simulink library "customLib"  (R2021b)
settings: Solver=VariableStepAuto  StartTime=0.0  StopTime=10.0  RelTol=1e-3
undefined symbols (not defined in the file or in its folder): D1, Delta
libraries: eeGeneralControl x7, spsParallelRLCBranchLib x6, spsSeriesRLCBranchLib x3, slpidlib x2, spsThreePhaseTransformerTwoWindingsLib x1
settings Model: Creator=ah4430  LastModifiedBy=ah4430

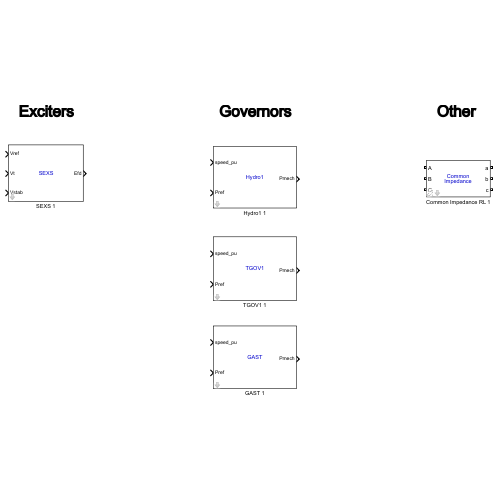
[thumbnail: Simulink's stored preview of the top-level diagram]
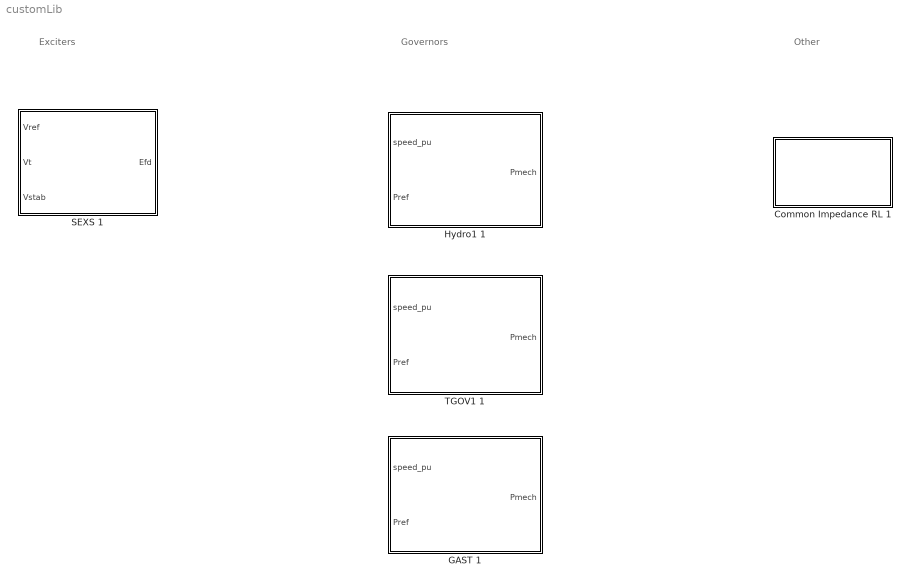
== system customLib ==
  note: Exciters
  note: Governors
  note: Other
  Common Impedance RL 1 : Subsystem  AncestorBlock=customLib/Common Impedance 1  mask{R=0.001, L=0, C=0, Ui=0, Ri=1e3, Li=1e-3, Uj=0, Rj=1e3, Lj=1e-3, Winding1Connection=Delta (D1), Winding2Connection=Delta (D1), ConnectionVariant=abc}
      mask prompts: R "Resistance [Ohm]"; L "Inductance [H]"; C "Capacitance [F]"; Ui "Voltage i [V]"; Ri "Resistance i [Ohm]"; Li "Inductance i [H]"; Uj "Voltage j [V]"; Rj "Resistance j [Ohm]"; Lj "Inductance j [H]"; Winding1Connection "Winding 1 connection (ABC terminals):"; Winding2Connection "Winding 2 connection (abc terminals):"; ConnectionVariant "Connection (abc, bca, cab)"
      mask TypeOptions Winding1Connection: Transformer/Winding1Connection
      mask TypeOptions Winding2Connection: Transformer/Winding2Connection
      mask TypeOptions ConnectionVariant: Connection/LabelModeActiveChoice
      mask Display: color('blue');disp('Common\nImpedance')
  GAST 1 : Subsystem  mask{R=0.05, T_1=0.2, T_2=0.2, T_3=1, A_T=0.5, K_T=1, Vmax=1.1, Vmin=0, DTurb=0}
      mask prompts: R "Permanent droop R (pu)"; T_1 "Governor mechanism time constant T_1 (s)"; T_2 "Turbine power time constant T_2 (s)"; T_3 "Turbine exhaust temperature time constant T_3 (s)"; A_T "Ambient temperature load limit A_T (pu)"; K_T "Temperature limiter gain K_T (pu)"; Vmax "Maximum turbine power Vmax (pu)"; Vmin "Minimum turbine power Vmin (pu)"; DTurb "Turbine damping factor DTurb (pu)"
      mask Display: color('blue');disp('GAST')
  Hydro1 1 : Subsystem  mask{Rt=0.3, TR=5, TF=0.05, TG=0.5, TW=1, AT=10, DT=0.5, QNL=0.08, Rp=0.29, Gmin=0, Gmax=1, Velm=0.2}
      mask prompts: Rt "Temporary droop Rt (pu)"; TR "Governor time constant TR (s)"; TF "Filter time constant TF (s)"; TG "Servo time constant TG (s)"; TW "Water starting time TW (s)"; AT "Turbine gain AT (pu)"; DT "Turbine damping factor DT (pu)"; QNL "No load flow QNL (pu)"; Rp "Permanent droop Rp (pu)"; Gmin "Minimum gate limit Gmin (pu)"; Gmax "Maximum gate limit Gmax (pu)"; Velm "Gate velocity limit Velm (pu)"
      mask Display: color('blue');disp('Hydro1')
  SEXS 1 : Subsystem  mask{TA=0, TB=0, K=0, TE=0, Emin=0, Emax=0}
      mask prompts: TA "Filter lead time constant TA (s)"; TB "Filter lag time constant TB (s)"; K "Controller gain K (pu)"; TE "Exciter time constant TE (s)"; Emin "Exciter minimum output Emin (pu)"; Emax "Exciter maximum output Emax (pu)"
      mask Display: color('blue');disp('SEXS')
  TGOV1 1 : Subsystem  mask(Governor TGOV1){R=0.05, T_1=0.2, Vmax=1.2, Vmin=0, T_2=1, T_3=3, Dt=0}
      mask prompts: R "Permanent droop R (pu)"; T_1 "Steam bowl time constant T_1 (s)"; Vmax "Maximum valve position Vmax (pu)"; Vmin "Minimum valve position Vmin (pu)"; T_2 "Time constant of high-pressure fraction T_2 (s)"; T_3 "Reheater time constant T_3 (s)"; Dt "Turbine damping coefficient Dt (pu)"
      mask help: Implements a TGOV1 governor.
      mask Display: color('blue');disp('TGOV1')

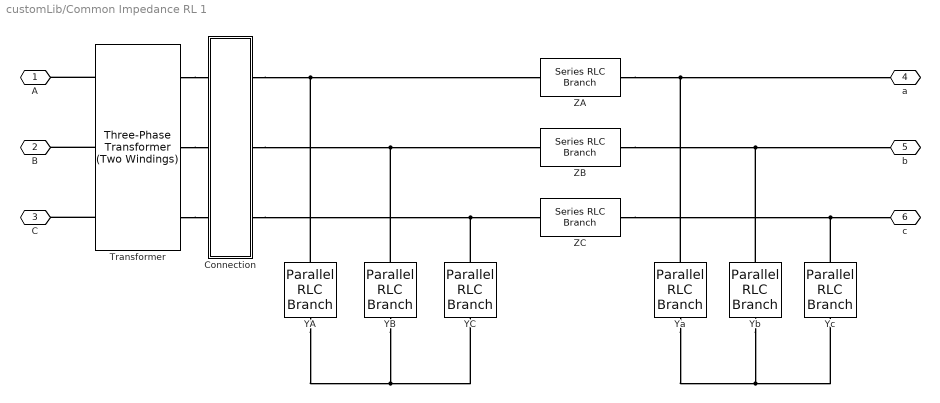
== system customLib/Common Impedance RL 1 ==
  Connection : Subsystem  Variant=on  VariantControlMode=label  LabelModeActiveChoice=abc
  Transformer : spsThreePhaseTransformerTwoWindingsLib/Three-Phase Transformer (Two Windings)  VariantControl=(default)  Winding1Connection=Delta (D1)  Winding2Connection=Delta (D1)  CoreType=Three single-phase transformers  SetSaturation=off  Hysteresis=off  DataFile='hysteresis'  SetInitialFlux=off  Measurements=None  UNITS=pu  NominalPower=[ 1e12 , 60 ]  Winding1=[Ui 1e-7 0]  Winding2=[Uj 1e-7 0]  Rm=1e7  Lm=1e7  L0=NaN  Saturation=[NaN NaN;NaN NaN;NaN NaN]  InitialFluxes=[NaN NaN NaN]  BreakLoop=off  DiscreteSolver=Trapezoidal iterative  DataType=off  TransfoNumber=1
  YA : spsParallelRLCBranchLib/Parallel RLC Branch  LConnTagsString=a  RConnTagsString=__new0  BranchType=RL  Resistance=Ri  Inductance=Li  SetiL0=off  InitialCurrent=0  Capacitance=1e-6  Setx0=off  InitialVoltage=0  Measurements=None
  YB : spsParallelRLCBranchLib/Parallel RLC Branch  LConnTagsString=a  RConnTagsString=__new0  BranchType=RL  Resistance=Ri  Inductance=Li  SetiL0=off  InitialCurrent=0  Capacitance=1e-6  Setx0=off  InitialVoltage=0  Measurements=None
  YC : spsParallelRLCBranchLib/Parallel RLC Branch  LConnTagsString=a  RConnTagsString=__new0  BranchType=RL  Resistance=Ri  Inductance=Li  SetiL0=off  InitialCurrent=0  Capacitance=1e-6  Setx0=off  InitialVoltage=0  Measurements=None
  Ya : spsParallelRLCBranchLib/Parallel RLC Branch  LConnTagsString=a  RConnTagsString=__new0  BranchType=RL  Resistance=Rj  Inductance=Lj  SetiL0=off  InitialCurrent=0  Capacitance=1e-6  Setx0=off  InitialVoltage=0  Measurements=None
  Yb : spsParallelRLCBranchLib/Parallel RLC Branch  LConnTagsString=a  RConnTagsString=__new0  BranchType=RL  Resistance=Rj  Inductance=Lj  SetiL0=off  InitialCurrent=0  Capacitance=1e-6  Setx0=off  InitialVoltage=0  Measurements=None
  Yc : spsParallelRLCBranchLib/Parallel RLC Branch  LConnTagsString=a  RConnTagsString=__new0  BranchType=RL  Resistance=Rj  Inductance=Lj  SetiL0=off  InitialCurrent=0  Capacitance=1e-6  Setx0=off  InitialVoltage=0  Measurements=None
  ZA : spsSeriesRLCBranchLib/Series RLC Branch  LConnTagsString=__new0  RConnTagsString=__new0  BranchType=RL  Resistance=R  Inductance=L  SetiL0=off  InitialCurrent=0  Capacitance=C  Setx0=off  InitialVoltage=0  Measurements=None
  ZB : spsSeriesRLCBranchLib/Series RLC Branch  LConnTagsString=__new0  RConnTagsString=__new0  BranchType=RL  Resistance=R  Inductance=L  SetiL0=off  InitialCurrent=0  Capacitance=C  Setx0=off  InitialVoltage=0  Measurements=None
  ZC : spsSeriesRLCBranchLib/Series RLC Branch  LConnTagsString=__new0  RConnTagsString=__new0  BranchType=RL  Resistance=R  Inductance=L  SetiL0=off  InitialCurrent=0  Capacitance=C  Setx0=off  InitialVoltage=0  Measurements=None
  A : PMIOPort  Side=Left
  B : PMIOPort  Port=2  Side=Left
  C : PMIOPort  Port=3  Side=Left
  a : PMIOPort  Port=4  Side=Right
  b : PMIOPort  Port=5  Side=Right
  c : PMIOPort  Port=6  Side=Right
  connections:
  YA/LConn1 -- ZA/LConn1 -- Connection/LConn1
  YC/LConn1 -- ZC/LConn1 -- Connection/LConn3
  YB/LConn1 -- ZB/LConn1 -- Connection/LConn2
  Ya/LConn1 -- ZA/RConn1 -- a/RConn1
  Yb/LConn1 -- ZB/RConn1 -- b/RConn1
  Yc/LConn1 -- ZC/RConn1 -- c/RConn1
  Transformer/LConn1 -- A/RConn1
  Transformer/LConn2 -- B/RConn1
  Transformer/LConn3 -- C/RConn1
  Ya/RConn1 -- Yb/RConn1 -- Yc/RConn1
  Transformer/RConn1 -- Connection/RConn1
  Transformer/RConn2 -- Connection/RConn2
  Transformer/RConn3 -- Connection/RConn3
  YB/RConn1 -- YC/RConn1 -- YA/RConn1

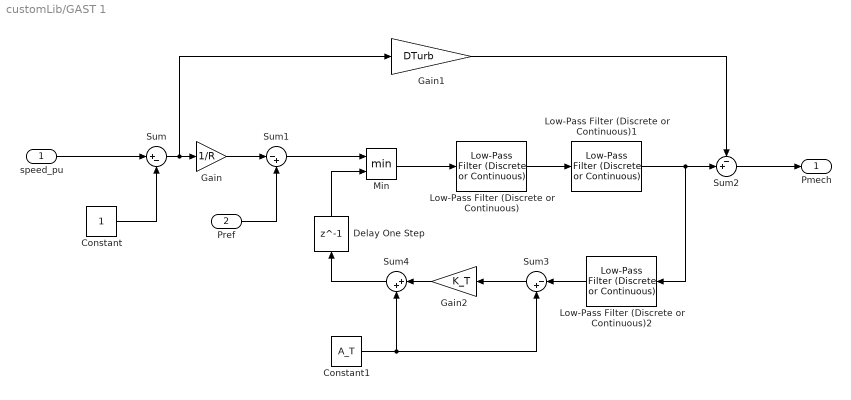
== system customLib/GAST 1 ==
  speed_pu : Inport
  Pref : Inport  Port=2
  Constant : Constant
  Constant1 : Constant  Value=A_T
  Delay One Step : Delay  DelayLength=1
  Gain : Gain  Gain=1/R
  Gain1 : Gain  Gain=DTurb
  Gain2 : Gain  Gain=K_T
  Low-Pass Filter (Discrete or Continuous) : eeGeneralControl/Low-Pass Filter (Discrete or Continuous)  K=1  T=T_1  B=Vmax  A=Vmin  init_option=Inherited from block input  x0=0  Ts=-1
  Low-Pass Filter (Discrete or Continuous)1 : eeGeneralControl/Low-Pass Filter (Discrete or Continuous)  K=1  T=T_2  B=inf  A=-inf  init_option=Inherited from block input  x0=0  Ts=-1
  Low-Pass Filter (Discrete or Continuous)2 : eeGeneralControl/Low-Pass Filter (Discrete or Continuous)  K=1  T=T_3  B=inf  A=-inf  init_option=Inherited from block input  x0=0  Ts=-1
  Min : MinMax  Inputs=2
  Sum : Sum  Inputs=|+-
  Sum1 : Sum  Inputs=|-+
  Sum2 : Sum  Inputs=-+|
  Sum3 : Sum  Inputs=|-+
  Sum4 : Sum  Inputs=|++
  Pmech : Outport
  wires:
  speed_pu/1 -> Sum/1
  Constant/1 -> Sum/2
  Sum/1 -> Gain1/1, Gain/1
  Gain/1 -> Sum1/1
  Pref/1 -> Sum1/2
  Sum1/1 -> Min/1
  Min/1 -> Low-Pass Filter (Discrete or Continuous)/1
  Low-Pass Filter (Discrete or Continuous)/1 -> Low-Pass Filter (Discrete or Continuous)1/1
  Low-Pass Filter (Discrete or Continuous)1/1 -> Low-Pass Filter (Discrete or Continuous)2/1, Sum2/2
  Gain1/1 -> Sum2/1
  Sum2/1 -> Pmech/1
  Low-Pass Filter (Discrete or Continuous)2/1 -> Sum3/1
  Constant1/1 -> Sum4/2, Sum3/2
  Sum3/1 -> Gain2/1
  Gain2/1 -> Sum4/1
  Sum4/1 -> Delay One Step/1
  Delay One Step/1 -> Min/2

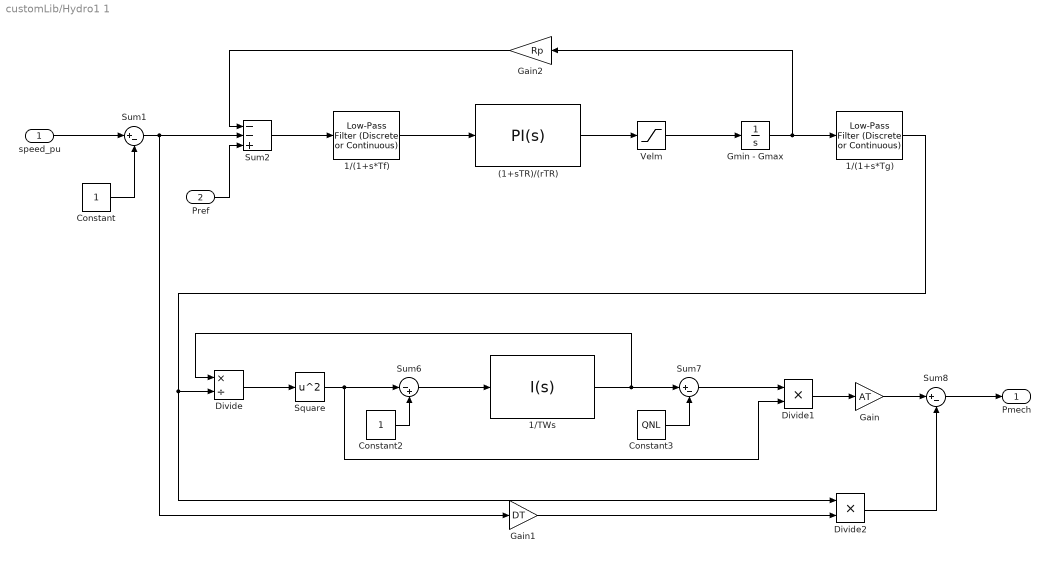
== system customLib/Hydro1 1 ==
  speed_pu : Inport
  Pref : Inport  Port=2
  (1+sTR)/(rTR) : slpidlib/PID Controller  Controller=PI  Form=Parallel  TimeDomain=Continuous-time  UseExternalTs=off  SampleTime=-1  IntegratorMethod=Forward Euler  FilterMethod=Forward Euler  ControllerParametersSource=internal  P=1/Rt  I=1/(Rt*TR)  D=0  UseFilter=on  N=100  TunerSelectOption=Transfer Function Based (PID Tuner App)  InitialConditionSource=internal  InitialConditionForIntegrator=0  InitialConditionForFilter=0  DifferentiatorICPrevScaledInput=0  ExternalReset=none  TrackingMode=off  Kt=1  LimitOutput=on  SatLimitsSource=internal  UpperSaturationLimit=Gmax  LowerSaturationLimit=Gmin  LinearizeAsGain=on  AntiWindupMode=none  Kb=1  POutMin=[]  POutMax=[]  IOutMin=[]  IOutMax=[]  DOutMin=[]  DOutMax=[]  NOutMin=[]  NOutMax=[]  SumOutMin=[]  SumOutMax=[]  SaturationOutMin=[]  SaturationOutMax=[]  PParamMin=[]  PParamMax=[]  IParamMin=[]  IParamMax=[]  DParamMin=[]  DParamMax=[]  NParamMin=[]  NParamMax=[]  KbParamMin=[]  KbParamMax=[]  KtParamMin=[]  KtParamMax=[]  KbOutMin=[]  KbOutMax=[]  KtOutMin=[]  KtOutMax=[]  IntegratorOutMin=[]  IntegratorOutMax=[]  FilterOutMin=[]  FilterOutMax=[]  SumI1OutMin=[]  SumI1OutMax=[]  SumI2OutMin=[]  SumI2OutMax=[]  SumI3OutMin=[]  SumI3OutMax=[]  SumI4OutMin=[]  SumI4OutMax=[]  SumDOutMin=[]  SumDOutMax=[]  DifferentiatorOutMin=[]  DifferentiatorOutMax=[]  FilterDiffOutCoefMin=[]  FilterDiffOutCoefMax=[]  ReciprocalOutMin=[]  ReciprocalOutMax=[]  SumDenOutMin=[]  SumDenOutMax=[]  SumNumOutMin=[]  SumNumOutMax=[]  DivideOutMin=[]  DivideOutMax=[]  UdiffTsProdOutMin=[]  UdiffTsProdOutMax=[]  NTsProdOutMin=[]  NTsProdOutMax=[]  UintegralTsProdOutMin=[]  UintegralTsProdOutMax=[]  UngainTsProdOutMin=[]  UngainTsProdOutMax=[]  FilterDenConstantOutDataTypeStr=Inherit: Inherit via back propagation  FilterDenConstantOutMin=[]  FilterDenConstantOutMax=[]  PCopyOutDataTypeStr=Inherit: Inherit via back propagation  PCopyOutMin=[]  PCopyOutMax=[]  NCopyOutDataTypeStr=Inherit: Inherit via back propagation  NCopyOutMin=[]  NCopyOutMax=[]  IntegratorContinuousStateAttributes=''  IntegratorStateMustResolveToSignalObject=off  IntegratorRTWStateStorageClass=Auto  FilterContinuousStateAttributes=''  FilterStateMustResolveToSignalObject=off  FilterRTWStateStorageClass=Auto  ParallelPVariant=InternalParameters  IdealPVariant=Disabled  IVariant=InternalParameters  DVariant=Disabled  IntegratorVariant=Continuous  SatVariant=Enabled  AWVariant=Passthrough  PCopyVariant=Disabled  TRVariant=Disabled  FdbkBlocksVariant=Forward  IdealPFdbkVariant=Disabled  SatFdbkVariant=Disabled  DerivativeFilterVariant=Disabled  NVariant=Disabled  NCopyVariant=Disabled_SignalSpec  FilterICVariant=Disabled  IntegratorICVariant=InternalICs  ExternalResetVariant=Disabled  TRSumVariant=Passthrough  SumFdbkVariant=Disabled  SumVariant=Sum_PI  TsampFilterVariant=InternalTs  TsampNgainVariant=Passthrough  TsampIntegralVariant=Passthrough  ExternalSaturationOutDataTypeStr=Inherit: Same as second input
  1/(1+s*Tf) : eeGeneralControl/Low-Pass Filter (Discrete or Continuous)  K=1  T=TF  B=inf  A=-inf  init_option=Inherited from block input  x0=0  Ts=-1
  1/(1+s*Tg) : eeGeneralControl/Low-Pass Filter (Discrete or Continuous)  K=1  T=TG  B=inf  A=-inf  init_option=Inherited from block input  x0=0  Ts=-1
  1/TWs : slpidlib/PID Controller  Controller=I  Form=Parallel  TimeDomain=Continuous-time  UseExternalTs=off  SampleTime=-1  IntegratorMethod=Forward Euler  FilterMethod=Forward Euler  ControllerParametersSource=internal  P=1  I=1/TW  D=0  UseFilter=on  N=100  TunerSelectOption=Transfer Function Based (PID Tuner App)  InitialConditionSource=internal  InitialConditionForIntegrator=0  InitialConditionForFilter=0  DifferentiatorICPrevScaledInput=0  ExternalReset=none  TrackingMode=off  Kt=1  LimitOutput=on  SatLimitsSource=internal  UpperSaturationLimit=Gmax  LowerSaturationLimit=Gmin  LinearizeAsGain=on  AntiWindupMode=none  Kb=1  POutMin=[]  POutMax=[]  IOutMin=[]  IOutMax=[]  DOutMin=[]  DOutMax=[]  NOutMin=[]  NOutMax=[]  SumOutMin=[]  SumOutMax=[]  SaturationOutMin=[]  SaturationOutMax=[]  PParamMin=[]  PParamMax=[]  IParamMin=[]  IParamMax=[]  DParamMin=[]  DParamMax=[]  NParamMin=[]  NParamMax=[]  KbParamMin=[]  KbParamMax=[]  KtParamMin=[]  KtParamMax=[]  KbOutMin=[]  KbOutMax=[]  KtOutMin=[]  KtOutMax=[]  IntegratorOutMin=[]  IntegratorOutMax=[]  FilterOutMin=[]  FilterOutMax=[]  SumI1OutMin=[]  SumI1OutMax=[]  SumI2OutMin=[]  SumI2OutMax=[]  SumI3OutMin=[]  SumI3OutMax=[]  SumI4OutMin=[]  SumI4OutMax=[]  SumDOutMin=[]  SumDOutMax=[]  DifferentiatorOutMin=[]  DifferentiatorOutMax=[]  FilterDiffOutCoefMin=[]  FilterDiffOutCoefMax=[]  ReciprocalOutMin=[]  ReciprocalOutMax=[]  SumDenOutMin=[]  SumDenOutMax=[]  SumNumOutMin=[]  SumNumOutMax=[]  DivideOutMin=[]  DivideOutMax=[]  UdiffTsProdOutMin=[]  UdiffTsProdOutMax=[]  NTsProdOutMin=[]  NTsProdOutMax=[]  UintegralTsProdOutMin=[]  UintegralTsProdOutMax=[]  UngainTsProdOutMin=[]  UngainTsProdOutMax=[]  FilterDenConstantOutDataTypeStr=Inherit: Inherit via back propagation  FilterDenConstantOutMin=[]  FilterDenConstantOutMax=[]  PCopyOutDataTypeStr=Inherit: Inherit via back propagation  PCopyOutMin=[]  PCopyOutMax=[]  NCopyOutDataTypeStr=Inherit: Inherit via back propagation  NCopyOutMin=[]  NCopyOutMax=[]  IntegratorContinuousStateAttributes=''  IntegratorStateMustResolveToSignalObject=off  IntegratorRTWStateStorageClass=Auto  FilterContinuousStateAttributes=''  FilterStateMustResolveToSignalObject=off  FilterRTWStateStorageClass=Auto  ParallelPVariant=Disabled  IdealPVariant=Disabled  IVariant=InternalParameters  DVariant=Disabled  IntegratorVariant=Continuous  SatVariant=Enabled  AWVariant=Passthrough  PCopyVariant=Disabled  TRVariant=Disabled  FdbkBlocksVariant=Forward  IdealPFdbkVariant=Disabled  SatFdbkVariant=Disabled  DerivativeFilterVariant=Disabled  NVariant=Disabled  NCopyVariant=Disabled_SignalSpec  FilterICVariant=Disabled  IntegratorICVariant=InternalICs  ExternalResetVariant=Disabled  TRSumVariant=Passthrough  SumFdbkVariant=Disabled  SumVariant=Passthrough_I  TsampFilterVariant=InternalTs  TsampNgainVariant=Passthrough  TsampIntegralVariant=Passthrough  ExternalSaturationOutDataTypeStr=Inherit: Same as second input
  Constant : Constant
  Constant2 : Constant
  Constant3 : Constant  Value=QNL
  Divide : Product  Inputs=*/
  Divide1 : Product
  Divide2 : Product
  Gain : Gain  Gain=AT
  Gain1 : Gain  Gain=DT
  Gain2 : Gain  Gain=Rp
  Gmin - Gmax : Integrator  LimitOutput=on  UpperSaturationLimit=Gmax  LowerSaturationLimit=Gmin
  Square : Math  Operator=square  SaturateOnIntegerOverflow=on
  Sum1 : Sum  Inputs=|+-
  Sum2 : Sum  Inputs=--+
  Sum6 : Sum  Inputs=|-+
  Sum7 : Sum  Inputs=|+-
  Sum8 : Sum  Inputs=|+-
  Velm : Saturate  UpperLimit=Velm  LowerLimit=-1 * Velm
  Pmech : Outport
  wires:
  Constant/1 -> Sum1/2
  speed_pu/1 -> Sum1/1
  Pref/1 -> Sum2/3
  Sum1/1 -> Sum2/2, Gain1/1
  Sum2/1 -> 1/(1+s*Tf)/1
  (1+sTR)/(rTR)/1 -> Velm/1
  1/(1+s*Tf)/1 -> (1+sTR)/(rTR)/1
  Velm/1 -> Gmin - Gmax/1
  Gmin - Gmax/1 -> 1/(1+s*Tg)/1, Gain2/1
  Gain2/1 -> Sum2/1
  1/(1+s*Tg)/1 -> Divide2/1, Divide/2
  Divide/1 -> Square/1
  Constant2/1 -> Sum6/2
  Square/1 -> Divide1/2, Sum6/1
  Sum6/1 -> 1/TWs/1
  1/TWs/1 -> Divide/1, Sum7/1
  Constant3/1 -> Sum7/2
  Sum7/1 -> Divide1/1
  Divide1/1 -> Gain/1
  Gain/1 -> Sum8/1
  Divide2/1 -> Sum8/2
  Gain1/1 -> Divide2/2
  Sum8/1 -> Pmech/1

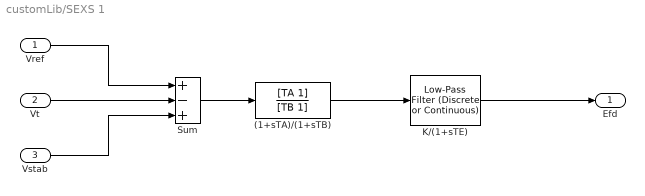
== system customLib/SEXS 1 ==
  Vref : Inport
  Vt : Inport  Port=2
  Vstab : Inport  Port=3
  (1+sTA)/(1+sTB) : TransferFcn  Numerator=[TA 1]  Denominator=[TB 1]
  K/(1+sTE) : eeGeneralControl/Low-Pass Filter (Discrete or Continuous)  K=K  T=TE  B=Emax  A=Emin  init_option=Inherited from block input  x0=0  Ts=-1
  Sum : Sum  Inputs=+-+
  Efd : Outport
  wires:
  Vref/1 -> Sum/1
  Vt/1 -> Sum/2
  Vstab/1 -> Sum/3
  Sum/1 -> (1+sTA)/(1+sTB)/1
  (1+sTA)/(1+sTB)/1 -> K/(1+sTE)/1
  K/(1+sTE)/1 -> Efd/1

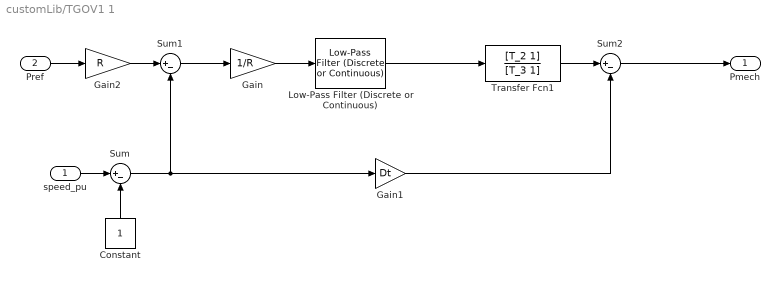
== system customLib/TGOV1 1 ==
  speed_pu : Inport
  Pref : Inport  Port=2
  Constant : Constant
  Gain : Gain  Gain=1/R
  Gain1 : Gain  Gain=Dt
  Gain2 : Gain  Gain=R
  Low-Pass Filter (Discrete or Continuous) : eeGeneralControl/Low-Pass Filter (Discrete or Continuous)  K=1  T=T_1  B=Vmax  A=Vmin  init_option=Inherited from block input  x0=0  Ts=-1
  Sum : Sum  Inputs=|+-
  Sum1 : Sum  Inputs=|+-
  Sum2 : Sum  Inputs=|+-
  Transfer Fcn1 : TransferFcn  Numerator=[T_2 1]  Denominator=[T_3 1]
  Pmech : Outport
  wires:
  Constant/1 -> Sum/2
  Gain1/1 -> Sum2/2
  Transfer Fcn1/1 -> Sum2/1
  Gain/1 -> Low-Pass Filter (Discrete or Continuous)/1
  Sum2/1 -> Pmech/1
  Sum/1 -> Gain1/1, Sum1/2
  speed_pu/1 -> Sum/1
  Sum1/1 -> Gain/1
  Low-Pass Filter (Discrete or Continuous)/1 -> Transfer Fcn1/1
  Pref/1 -> Gain2/1
  Gain2/1 -> Sum1/1

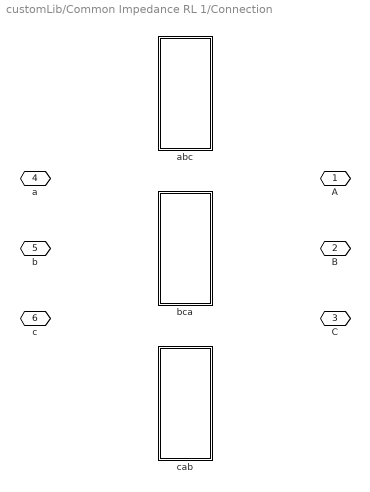
== system customLib/Common Impedance RL 1/Connection ==
  abc : Subsystem  VariantControl=abc
  bca : Subsystem  AncestorBlock=customLib/Common Impedance RL 1/Variant Subsystem/abc  VariantControl=bca
  cab : Subsystem  AncestorBlock=customLib/Common Impedance RL 1/Variant Subsystem/abc  VariantControl=cab
  A : PMIOPort  Side=Left
  B : PMIOPort  Port=2  Side=Left
  C : PMIOPort  Port=3  Side=Left
  a : PMIOPort  Port=4  Side=Right
  b : PMIOPort  Port=5  Side=Right
  c : PMIOPort  Port=6  Side=Right

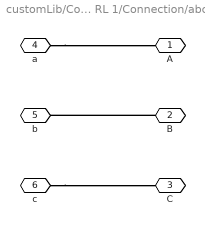
== system customLib/Common Impedance RL 1/Connection/abc ==
  A : PMIOPort  Side=Left
  B : PMIOPort  Port=2  Side=Left
  C : PMIOPort  Port=3  Side=Left
  a : PMIOPort  Port=4  Side=Right
  b : PMIOPort  Port=5  Side=Right
  c : PMIOPort  Port=6  Side=Right
  connections:
  B/RConn1 -- b/RConn1
  a/RConn1 -- A/RConn1
  c/RConn1 -- C/RConn1

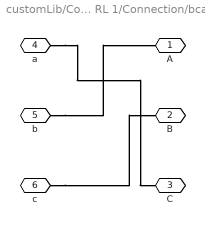
== system customLib/Common Impedance RL 1/Connection/bca ==
  A : PMIOPort  Side=Left
  B : PMIOPort  Port=2  Side=Left
  C : PMIOPort  Port=3  Side=Left
  a : PMIOPort  Port=4  Side=Right
  b : PMIOPort  Port=5  Side=Right
  c : PMIOPort  Port=6  Side=Right
  connections:
  b/RConn1 -- A/RConn1
  c/RConn1 -- B/RConn1
  a/RConn1 -- C/RConn1

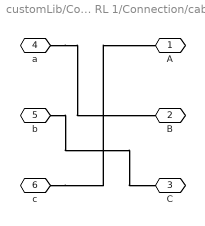
== system customLib/Common Impedance RL 1/Connection/cab ==
  A : PMIOPort  Side=Left
  B : PMIOPort  Port=2  Side=Left
  C : PMIOPort  Port=3  Side=Left
  a : PMIOPort  Port=4  Side=Right
  b : PMIOPort  Port=5  Side=Right
  c : PMIOPort  Port=6  Side=Right
  connections:
  c/RConn1 -- A/RConn1
  a/RConn1 -- B/RConn1
  b/RConn1 -- C/RConn1
